simulink model "WaterRunner_open"  (Simulink 8.0)
settings: Solver=ode15s  StartTime=0.0  StopTime=10  FixedStep=1e-3  RelTol=1e-3
values from neighbouring files (symbols this model uses):
  frame_inertia = diag([Ix,Iy,Iz])    [SimParam.m]    (also in matlab.mat = [8.0125e-05  0  0; 0  0.000390625  0; 0  0  0.0003145]; simParams.m; simParams_closed.m; speed_cg.mat = [8.0125e-05  0  0; 0  0.000390625  0; 0  0  0.0003145])
  frame_mass = 0.06    [matlab.mat]    (also in simParam.m = 0.03; simParams.m; simParams_closed.m = 0.1; speed_cg.mat)
  freq = 60    [SimParam.m]    (also in simParam.m = 20; simParams_closed.m)
  L2_inertia = [1.05087286587e-08  0  0; 0  0  0; 0  0  1.05087286587e-08]    [matlab.mat]    (also in simParams.m = diag([I 0 I]); simParams_closed.m = diag([I 0 I]); speed_cg.mat)
  L2_mass = 0.0002653496    [matlab.mat]    (also in simParams.m; simParams_closed.m; speed_cg.mat)
  L3_inertia = [4.24507620885e-07  0  0; 0  0  0; 0  0  4.24507620885e-07]    [matlab.mat]    (also in simParams.m = diag([I 0 I]); simParams_closed.m = diag([I 0 I]); speed_cg.mat)
  L3_mass = 0.0009104656    [matlab.mat]    (also in simParams.m; simParams_closed.m; speed_cg.mat)
  L4_inertia = [1.03972444992e-07  0  0; 0  0  0; 0  0  1.03972444992e-07]    [matlab.mat]    (also in simParams.m = diag([I 0 I]); simParams_closed.m = diag([I 0 I]); speed_cg.mat)
  L4_mass = 0.0005696496    [matlab.mat]    (also in simParams.m; simParams_closed.m; speed_cg.mat)
  water_level = 0    [matlab.mat]    (also in simParam.m; simParams.m; simParams_closed.m; speed_cg.mat)
undefined symbols (not defined in the file): cw_FL_HL, cw_FR_FL, cw_FR_HR, cw_HR_HL, FL_HL_lag, FR_FL_lag, FR_HR_lag, HR_HL_lag, initRobHeight
libraries: mblibv1 x17, WaterRunner_lib x14, simulink x1
settings Model: Creator=fumiyaiida  LastModifiedBy=nitisht  SimulationMode=accelerator
settings SolverCC: ZeroCrossControl=DisableAll
settings DataIOCC: SignalLoggingSaveFormat=ModelDataLogs
settings OptimizationCC: InlineInvariantSignals=on  InitFltsAndDblsToZero=on  EfficientMapNaN2IntZero=off  SimCompilerOptimization=On
settings DebuggingCC: SaveWithParameterizedLinksMsg=none  SignalResolutionControl=TryResolveAllWithWarning  SolverPrmCheckMsg=none  MultiTaskDSMMsg=warning  MultiTaskCondExecSysMsg=none  FcnCallInpInsideContextMsg=UseLocalSettings  StrictBusMsg=None
settings HardwareCC: ProdBitPerLong=64  ProdBitPerPointer=64  ProdIntDivRoundTo=Zero  ProdEndianess=LittleEndian  ProdWordSize=64  ProdHWDeviceType=Intel->x86-64  TargetBitPerLong=64  TargetBitPerPointer=64  TargetIntDivRoundTo=Zero  TargetEndianess=LittleEndian  TargetWordSize=64  TargetHWDeviceType=MATLAB Host  ProdEqTarget=off
settings RTWCC: RTWCompilerOptimization=On
settings CodeAppCC: MaxIdLength=128
settings GRTTargetCC: CombineOutputUpdateFcns=off  GRTInterface=on
settings SimMechanicsCC: WarnOnSingularInitialAssembly=on  VisDuringSimulation=on  VisSampleTime=0.001  AnimationDelay=1  LastVizWinPosition=[1323 2 597 976]  CamPosition=[-7.43826;3.54067;9.27536;]  CamTarget=[0.848137;-0.562095;-0.541519;]  CamUpVector=[0.217493;0.952228;-0.21438;]  CamHeight=2.55  VisBackgroundColor=[0.9;0.9;0.95;]  DefaultBodyColor=[1;0;0;]
settings ConfigurationSet: Description=SimMechanics 2G

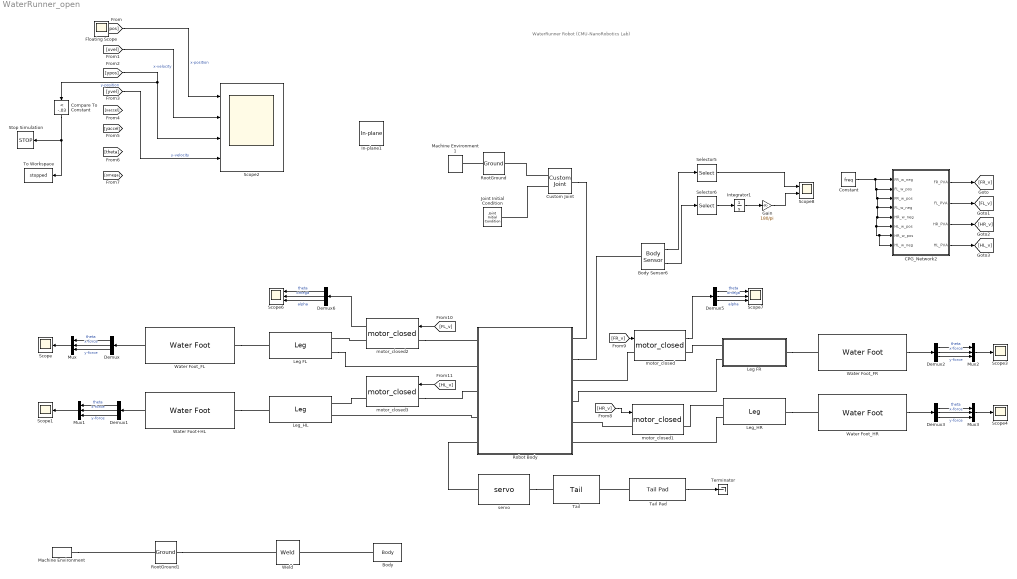
== system WaterRunner_open ==
  note: WaterRunner Robot
      | (CMU-NanoRobotics Lab)
  Body : mblibv1/Bodies/Body  LConnTagsString=CG  UpdateFromCAD=off  DialogClass=MechanicalBodyBlock  Mass=1  MassUnits=kg  InertiaUnits=kg*m^2  Inertia=eye(3)  Shape=Cylinder  ShapeDims=[1 1]  ShapeUnits=m  ShapeUse=false  Density=1  DensityUnits=kg/m^3  DensityUse=false  GraphicsMode=CONVHULL  BodyColorSelMode=COLORPALETTE  BodyColor=[0.83137 0.81569 0.78431]  AttachedToCS=CG  CG=Left$CG$[0 0 0]$WORLD$WORLD$m$[0 0 0]$Euler X-Y-Z$deg$WORLD$true$none  WorkingFrames=Left$CS1$[-0.5 water_level -0.2 ]$CG$CG$m$[0 0 0]$Euler X-Y-Z$deg$WORLD$false$none#Left$CS2$[-0.5 water_level 0.2 ]$CG$CG$m$[0 0 0]$Euler X-Y-Z$deg$WORLD$false$none#Left$CS3$[4 water_level -0.2 ]$CG$CG$m$[0 0 0]$Euler X-Y-Z$deg$WORLD$false$none#Left$CS4$[4 water_level 0.2 ]$CG$CG$m$[0 0 0]$Euler X-Y-Z$deg$WORLD$false$none  CGPos=[0 0 0]  CGRot=[0 0 0]  CS0Pos=[]  CS0Rot=[]  CS1Pos=[-0.5 water_level -0.2 ]  CS1Rot=[0 0 0]  CS2Pos=[-0.5 water_level 0.2 ]  CS2Rot=[0 0 0]  CS3Pos=[4 water_level -0.2 ]  CS3Rot=[0 0 0]  CS4Pos=[4 water_level 0.2 ]  CS4Rot=[0 0 0]  CS5Pos=[]  CS5Rot=[]  CS6Pos=[]  CS6Rot=[]  CS7Pos=[]  CS7Rot=[]  CS8Pos=[]  CS8Rot=[]  CS9Pos=[]  CS9Rot=[]  CS10Pos=[]  CS10Rot=[]  CS11Pos=[]  CS11Rot=[]  CS12Pos=[]  CS12Rot=[]  CS13Pos=[]  CS13Rot=[]  CS14Pos=[]  CS14Rot=[]  CS15Pos=[]  CS15Rot=[]  CS16Pos=[]  CS16Rot=[]  CS17Pos=[]  CS17Rot=[]  CS18Pos=[]  CS18Rot=[]  CS19Pos=[]  CS19Rot=[]  CS20Pos=[]  CS20Rot=[]
  Body Sensor6 : mblibv1/Sensors &  Actuators/Body Sensor  UpdateFromCAD=off  PhysicalDomain=Mechanical  PortType=blob  Muxed=off  Pose=off  Angle=on  AngleUnits=deg  ArcVelocity=on  ArcVelocityUnits=rad/s  ArcAcceleration=off  ArcAccelerationUnits=deg/s^2  CoordPosition=off  CoordPositionUnits=m  Velocity=on  VelocityUnits=m/s  Acceleration=off  AccelerationUnits=m/s^2  Quaternion=on  QuaternionDT=off  QuaternionDDT=off  QuaternionUnits=off  OutputVector=[1]  ActiveIO=on  Width=6  DialogClass=MechanicalSensorBlock  ReferenceFrame=Absolute (World)
  CPG_Network2 : Subsystem
  Compare To Constant : simulink/Logic and Bit Operations/Compare To Constant  relop=<  const=-.03  OutDataTypeStr=boolean
  Constant : Constant  Value=freq
  Custom Joint : mblibv1/Joints/Custom Joint  LConnTagsString=__newl0|SA1  RConnTagsString=__newr0  UpdateFromCAD=off  NumSAPorts=1  CutJoint=off  MarkAsCut=off  Primitives=prismatic  PrimitiveProps=P1$World$[0 1 0]$Prismatic#P2$World$[1 0 0]$Prismatic#R1$World$[0 0 1]$Revolute  DialogClass=JointBlock  R1Axis=[0 0 1]  R2Axis=[]  R3Axis=[]  P1Axis=[0 1 0]  P2Axis=[1 0 0]  P3Axis=[]  SAxis=[]
  Demux{,1..3,5..6} (6 alike) : Demux  Outputs=3
  Gain : Gain  Gain=180/pi
  In-plane1 : mblibv1/Joints/In-plane  LConnTagsString=__newl0|SA1|SA2  RConnTagsString=__newr0|SA1|SA2  UpdateFromCAD=off  NumSAPorts=4  CutJoint=off  MarkAsCut=off  Primitives=prismatic  PrimitiveProps=P1$World$[1 0 0]$prismatic#P2$World$[0 1 0]$prismatic  DialogClass=JointBlock  P1Axis=[1 0 0]  P2Axis=[0 1 0]
  Integrator1 : Integrator
  Joint Initial Condition : mblibv1/Sensors &  Actuators/Joint Initial Condition  UpdateFromCAD=off  LeftPortType=blob  RightPortType=blob  PhysicalDomain=mechanical  DialogClass=InitialConditionBlock  InitialConditions=P1$true$0$m$deg$0$m/s$deg/s#P2$true$initRobHeight$m$deg$0$m/s$deg/s#P3$false$0$m$deg$0$m/s$deg/s#R1$true$0$m$rad$0$m/s$rad/s#R2$false$0$m$deg$0$m/s$deg/s#R3$false$0$m$deg$0$m/s$deg/s#S$false$0$m$deg$0$m/s$deg/s  P1PIC=0  P1VIC=0  P2PIC=initRobHeight  P2VIC=0  P3PIC=0  P3VIC=0  R1PIC=0  R1VIC=0  R2PIC=0  R2VIC=0  R3PIC=0  R3VIC=0  SPIC=0  SVIC=0
  Leg FL : WaterRunner_lib/Leg
  Leg FR : Subsystem  AncestorBlock=WaterRunner_lib/Leg
      mask help: mask for leg
  Leg_HL : WaterRunner_lib/Leg
  Leg_HR : WaterRunner_lib/Leg
  Machine Environment : mblibv1/Bodies/Machine Environment  PortType=env  PhysicalDomain=Mechanical  DialogTemplateClass=MECH.MachineEnvironment  SyncWhenCopied=off  Gravity=[0 -9.81 0]  GravityUnits=m/s^2  GravityAsSignal=off  Dimensionality=Auto-detect  AnalysisType=Forward dynamics  LinearAssemblyTolerance=1e-3  LinearAssemblyToleranceUnits=m  AngularAssemblyTolerance=1e-3  AngularAssemblyToleranceUnits=rad  ConstraintSolverType=Stabilizing  ConstraintRelTolerance=1e-4  ConstraintAbsTolerance=1e-4  UseRobustSingularityHandling=off  RedundancyAnalysisToleranceType=Automatically select tolerance  RedundancyAnalysisTolerance=1e-14  StatePerturbationType=Fixed  PerturbationSize=1e-5  VisualizeMachine=on  BodyVisualizationType=Use model default body geometries  BodyColorSelMode=Use model default  DefaultBodyColor=[1 0 0]
  Machine Environment1 : mblibv1/Bodies/Machine Environment  PortType=env  PhysicalDomain=Mechanical  DialogTemplateClass=MECH.MachineEnvironment  SyncWhenCopied=off  Gravity=[0 -9.81 0]  GravityUnits=m/s^2  GravityAsSignal=off  Dimensionality=Auto-detect  AnalysisType=Forward dynamics  LinearAssemblyTolerance=1e-3  LinearAssemblyToleranceUnits=m  AngularAssemblyTolerance=1e-3  AngularAssemblyToleranceUnits=rad  ConstraintSolverType=Stabilizing  ConstraintRelTolerance=1e-4  ConstraintAbsTolerance=1e-4  UseRobustSingularityHandling=off  RedundancyAnalysisToleranceType=Automatically select tolerance  RedundancyAnalysisTolerance=1e-14  StatePerturbationType=Fixed  PerturbationSize=1e-5  VisualizeMachine=on  BodyVisualizationType=Use model default body geometries  BodyColorSelMode=Use model default  DefaultBodyColor=[1 0 0]
  Mux{,1..3} (4 alike) : Mux  Inputs=3
  Robot Body : Subsystem  AncestorBlock=WaterRunner_lib/Robot Body  mask{initRobHeight=initRobHeight}
      mask prompts: initRobHeight "height"
  RootGround : mblibv1/Bodies/Ground  UpdateFromCAD=on  LeftPortType=env  RightPortType=workingframe  PhysicalDomain=Mechanical  DialogClass=GroundBlock  CoordPosition=[0 0 0]  CoordPositionUnits=m  StateVectorMgrId=1  MachineId=[1 2]  ShowEnvPort=on
  RootGround1 : mblibv1/Bodies/Ground  UpdateFromCAD=on  LeftPortType=env  RightPortType=workingframe  PhysicalDomain=Mechanical  DialogClass=GroundBlock  CoordPosition=[0 0 0]  CoordPositionUnits=m  StateVectorMgrId=0  MachineId=[1 1]  ShowEnvPort=on
  Scope{,1,3..4} (4 alike) : Scope
      Scope settings: ShowLegends=on  TimeRange=2  YMin=-2.5  YMax=2  SaveName=FootForce_FL
      Scope1 settings: ShowLegends=on  TimeRange=2  YMin=-2.5  YMax=2  SaveName=FootForce_HL
      Scope3 settings: ShowLegends=on  TimeRange=2  YMin=-2.5  YMax=2  SaveName=FootForce_FR
      Scope4 settings: ShowLegends=on  TimeRange=2  YMin=-2.5  YMax=2  SaveName=FootForce_HR
  Scope2 : Scope  NumInputPorts=4
      settings: ShowLegends=on  TimeRange=10  YMin=-0.25~0~-0.005~-0.3  YMax=2~2.5~0.035~0.4  SaveName=position
  Scope6 : Scope  NumInputPorts=3
      settings: TimeRange=2  YMin=-20~-90~-50000  YMax=-2.5~0~30000  SaveName=MotorMotion1
  Scope7 : Scope  NumInputPorts=3
      settings: TimeRange=2  YMin=-17.5~-90~-70000  YMax=0~0~30000  SaveName=MotorMotion
  Scope8 : Scope  NumInputPorts=2
      settings: TimeRange=10  YMin=-0.15~0  YMax=0.225~20  SaveName=ball_position
  Selector5 : Selector  InputPortWidth=3  IndexOptions=Index vector (dialog)  Indices=[2]  OutputSizes=1
  Selector6 : Selector  InputPortWidth=3  IndexOptions=Index vector (dialog)  Indices=[1 3]  OutputSizes=1
  Stop Simulation : Stop
  Tail : WaterRunner_lib/Tail
  Tail Pad : WaterRunner_lib/Tail Pad
  Terminator : Terminator
  To Workspace : ToWorkspace  VariableName=stopped  SampleTime=-1  SaveFormat=Timeseries
  Water Foot+HL : WaterRunner_lib/Water Foot
  Water Foot_FL : WaterRunner_lib/Water Foot
  Water Foot_FR : WaterRunner_lib/Water Foot
  Water Foot_HR : WaterRunner_lib/Water Foot
  Weld : mblibv1/Joints/Weld  LConnTagsString=__newl0  RConnTagsString=__newr0  UpdateFromCAD=off  NumSAPorts=0  CutJoint=off  MarkAsCut=off  Primitives=weld  PrimitiveProps=W$WORLD$[0 0 0]$weld  DialogClass=JointBlock  WAxis=[0 0 0]
  motor_closed : WaterRunner_lib/motor_closed  ic_angle=pi
  motor_closed1 : WaterRunner_lib/motor_closed  ic_angle=0
  motor_closed2 : WaterRunner_lib/motor_closed  ic_angle=0
  motor_closed3 : WaterRunner_lib/motor_closed  ic_angle=pi
  servo : WaterRunner_lib/servo  tail_angle=tail_angle  VariableName=work_tail
  Floating Scope : Scope
      settings: Floating=on
  wires:
  Water Foot_FL/1 -> Demux/1
  Demux/1 -> Mux/1  "theta"
  Demux/2 -> Mux/2  "x-force"
  Demux/3 -> Mux/3  "y-force"
  Mux/1 -> Scope/1
  [ypos] -> Compare To Constant/1, Scope2/3  "y-position"
  Water Foot+HL/1 -> Demux1/1
  Demux1/1 -> Mux1/1  "theta"
  Demux1/2 -> Mux1/2  "x-force"
  Demux1/3 -> Mux1/3  "y-force"
  Mux1/1 -> Scope1/1
  Mux2/1 -> Scope3/1
  Demux2/3 -> Mux2/3  "y-force"
  Demux2/2 -> Mux2/2  "x-force"
  Demux2/1 -> Mux2/1  "theta"
  Water Foot_FR/1 -> Demux2/1
  Mux3/1 -> Scope4/1
  Demux3/3 -> Mux3/3  "y-force"
  Demux3/2 -> Mux3/2  "x-force"
  Demux3/1 -> Mux3/1  "theta"
  Water Foot_HR/1 -> Demux3/1
  Compare To Constant/1 -> To Workspace/1, Stop Simulation/1
  Demux5/3 -> Scope7/3  "alpha"
  Demux5/2 -> Scope7/2  "omega"
  Demux5/1 -> Scope7/1  "theta"
  motor_closed/1 -> Demux5/1
  Demux6/3 -> Scope6/3  "alpha"
  Demux6/2 -> Scope6/2  "omega"
  Demux6/1 -> Scope6/1  "theta"
  motor_closed2/1 -> Demux6/1
  Tail Pad/1 -> Terminator/1
  [xpos] -> Scope2/1  "x-position"
  [xvel] -> Scope2/2  "x-velocity"
  [yvel] -> Scope2/4  "y-velocity"
  CPG_Network2/1(FR_PVA) -> [FR_v]
  CPG_Network2/2(FL_PVA) -> [FL_v]
  CPG_Network2/3(HR_PVA) -> [HR_v]
  CPG_Network2/4(HL_PVA) -> [HL_v]
  [FR_v] -> motor_closed/1
  [HR_v] -> motor_closed1/1
  [FL_v] -> motor_closed2/1
  [HL_v] -> motor_closed3/1
  Selector6/1 -> Integrator1/1
  Body Sensor6/2 -> Selector6/1
  Integrator1/1 -> Gain/1
  Gain/1 -> Scope8/2
  Body Sensor6/1 -> Selector5/1
  Selector5/1 -> Scope8/1
  Constant/1 -> CPG_Network2/8(HL_w_neg), CPG_Network2/7(HR_w_pos), CPG_Network2/6(HL_w_pos), CPG_Network2/5(HR_w_neg), CPG_Network2/4(FL_w_neg), CPG_Network2/3(FR_w_pos), CPG_Network2/2(FL_w_pos), CPG_Network2/1(FR_w_neg)
  connections:
  RootGround1/RConn1 -- Weld/LConn1
  Body/LConn1 -- Weld/RConn1
  motor_closed/LConn1 -- Robot Body/RConn3
  Leg FR/LConn2 -- Robot Body/RConn4
  motor_closed/RConn1 -- Leg FR/LConn1
  motor_closed1/LConn1 -- Robot Body/RConn5
  motor_closed1/RConn1 -- Leg_HR/LConn1
  Leg_HR/LConn2 -- Robot Body/RConn6
  Water Foot+HL/LConn1 -- Leg_HL/RConn1
  Water Foot_FL/LConn1 -- Leg FL/RConn1
  Robot Body/LConn4 -- Leg_HL/LConn2
  Leg FR/RConn1 -- Water Foot_FR/LConn1
  Leg_HR/RConn1 -- Water Foot_HR/LConn1
  motor_closed2/LConn1 -- Robot Body/LConn1
  motor_closed3/RConn1 -- Leg_HL/LConn1
  motor_closed3/LConn1 -- Robot Body/LConn3
  Leg FL/LConn2 -- Robot Body/LConn2
  Machine Environment/RConn1 -- RootGround1/LConn1
  motor_closed2/RConn1 -- Leg FL/LConn1
  Robot Body/LConn5 -- servo/LConn1
  servo/RConn1 -- Tail/LConn1
  Tail Pad/LConn1 -- Tail/RConn1
  Custom Joint/LConn1 -- RootGround/RConn1
  Custom Joint/LConn2 -- Joint Initial Condition/RConn1
  RootGround/LConn1 -- Machine Environment1/RConn1
  Robot Body/RConn2 -- Body Sensor6/LConn1
  Custom Joint/RConn1 -- Robot Body/RConn1

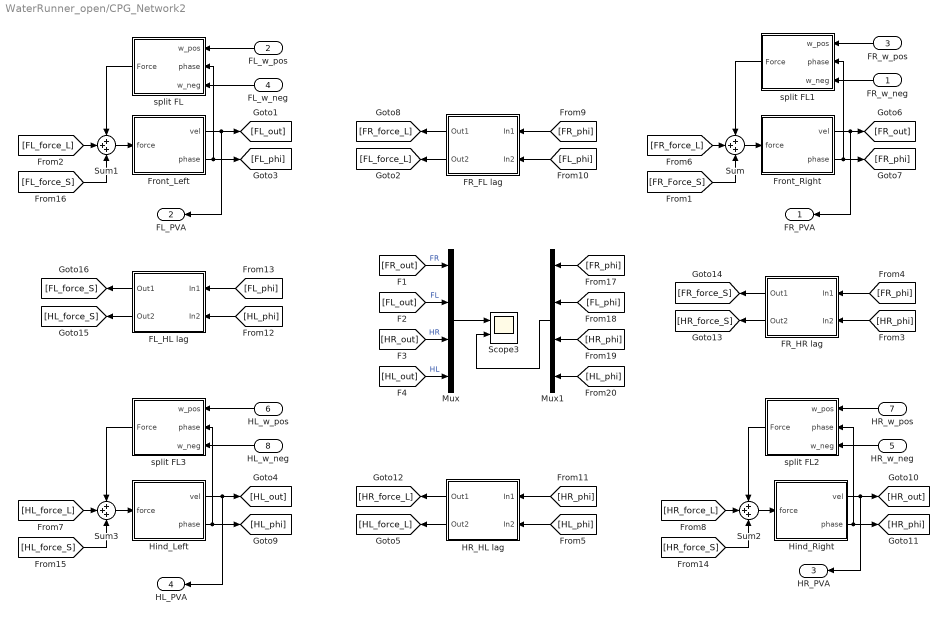
== system WaterRunner_open/CPG_Network2 ==
  FR_w_neg : Inport
  FL_w_pos : Inport  Port=2
  FR_w_pos : Inport  Port=3
  FL_w_neg : Inport  Port=4
  HR_w_neg : Inport  Port=5
  HL_w_pos : Inport  Port=6
  HR_w_pos : Inport  Port=7
  HL_w_neg : Inport  Port=8
  FL_HL lag : Subsystem  mask{d_phase=FL_HL_lag, coupling_weight=cw_FL_HL}
      mask prompts: d_phase "Phase Lag"; coupling_weight "Coupling Weight"
  FR_FL lag : Subsystem  mask{d_phase=FR_FL_lag, coupling_weight=cw_FR_FL}
      mask prompts: d_phase "Phase Lag"; coupling_weight "Coupling Weight"
  FR_HR lag : Subsystem  mask{d_phase=FR_HR_lag, coupling_weight=cw_FR_HR}
      mask prompts: d_phase "Phase Lag"; coupling_weight "Coupling Weight"
  Front_Left : Subsystem  mask{init_phi=0}
      mask prompts: init_phi "Initial Phase"
  Front_Right : Subsystem  mask{init_phi=pi}
      mask prompts: init_phi "Initial Phase"
  HR_HL lag : Subsystem  mask{d_phase=HR_HL_lag, coupling_weight=cw_HR_HL}
      mask prompts: d_phase "Phase Lag"; coupling_weight "Coupling Weight"
  Hind_Left : Subsystem  mask{init_phi=pi}
      mask prompts: init_phi "Initial Phase"
  Hind_Right : Subsystem  mask{init_phi=0}
      mask prompts: init_phi "Initial Phase"
  Mux : Mux
  Mux1 : Mux
  Scope3 : Scope  NumInputPorts=2
      settings: ShowLegends=on  TimeRange=5  YMin=22.11~0  YMax=22.34~6.5  SaveName=Output
  Sum{,1..3} (4 alike) : Sum  Inputs=+++
  split FL : Subsystem
  split FL1 : Subsystem
  split FL2 : Subsystem
  split FL3 : Subsystem
  FR_PVA : Outport
  FL_PVA : Outport  Port=2
  HR_PVA : Outport  Port=3
  HL_PVA : Outport  Port=4
  wires:
  Mux/1 -> Scope3/1
  Front_Left/2(phase) -> split FL/2(phase), [FL_phi]
  Front_Right/2(phase) -> split FL1/2(phase), [FR_phi]
  [FL_phi] -> FR_FL lag/2(In2)
  [FR_phi] -> FR_FL lag/1(In1)
  FR_FL lag/1(Out1) -> [FR_force_L]
  FR_FL lag/2(Out2) -> [FL_force_L]
  Front_Right/1(vel) -> FR_PVA/1, [FR_out]
  [FL_force_L] -> Sum1/2
  Sum1/1 -> Front_Left/1(force)
  Sum/1 -> Front_Right/1(force)
  [FR_force_L] -> Sum/2
  [FL_out] -> Mux/2  "FL"
  [FR_out] -> Mux/1  "FR"
  FR_w_pos/1 -> split FL1/1(w_pos)
  FR_w_neg/1 -> split FL1/3(w_neg)
  split FL1/1(Force) -> Sum/1
  FL_w_pos/1 -> split FL/1(w_pos)
  FL_w_neg/1 -> split FL/3(w_neg)
  Front_Left/1(vel) -> FL_PVA/1, [FL_out]
  split FL/1(Force) -> Sum1/1
  Hind_Left/2(phase) -> split FL3/2(phase), [HL_phi]
  Hind_Right/2(phase) -> [HR_phi], split FL2/2(phase)
  [HL_phi] -> HR_HL lag/2(In2)
  [HR_phi] -> HR_HL lag/1(In1)
  HR_HL lag/1(Out1) -> [HR_force_L]
  HR_HL lag/2(Out2) -> [HL_force_L]
  Hind_Right/1(vel) -> HR_PVA/1, [HR_out]
  [HL_force_L] -> Sum3/2
  Sum3/1 -> Hind_Left/1(force)
  Sum2/1 -> Hind_Right/1(force)
  [HR_force_L] -> Sum2/2
  HR_w_pos/1 -> split FL2/1(w_pos)
  HR_w_neg/1 -> split FL2/3(w_neg)
  split FL2/1(Force) -> Sum2/1
  HL_w_pos/1 -> split FL3/1(w_pos)
  HL_w_neg/1 -> split FL3/3(w_neg)
  Hind_Left/1(vel) -> HL_PVA/1, [HL_out]
  split FL3/1(Force) -> Sum3/1
  [HR_phi] -> FR_HR lag/2(In2)
  [FR_phi] -> FR_HR lag/1(In1)
  FR_HR lag/1(Out1) -> [FR_force_S]
  FR_HR lag/2(Out2) -> [HR_force_S]
  [HL_phi] -> FL_HL lag/2(In2)
  [FL_phi] -> FL_HL lag/1(In1)
  FL_HL lag/1(Out1) -> [FL_force_S]
  FL_HL lag/2(Out2) -> [HL_force_S]
  [HL_out] -> Mux/4  "HL"
  [HR_out] -> Mux/3  "HR"
  [FR_Force_S] -> Sum/3
  [HR_force_S] -> Sum2/3
  [HL_force_S] -> Sum3/3
  [FL_force_S] -> Sum1/3
  Mux1/1 -> Scope3/2
  [FR_phi] -> Mux1/1
  [FL_phi] -> Mux1/2
  [HR_phi] -> Mux1/3
  [HL_phi] -> Mux1/4

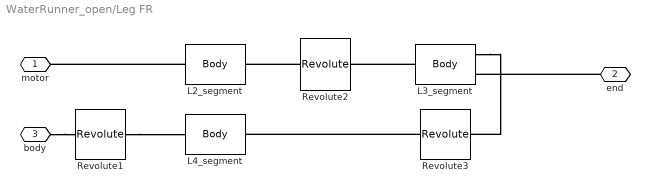
== system WaterRunner_open/Leg FR ==
  L2_segment : mblibv1/Bodies/Body  LConnTagsString=CS1  RConnTagsString=CS2  UpdateFromCAD=off  DialogClass=MechanicalBodyBlock  Mass=L2_mass  MassUnits=kg  InertiaUnits=kg*m^2  Inertia=L2_inertia  Shape=Cylinder  ShapeDims=[1 1]  ShapeUnits=m  ShapeUse=false  Density=1  DensityUnits=kg/m^3  DensityUse=false  GraphicsMode=CONVHULL  BodyColorSelMode=COLORPALETTE  BodyColor=[0 0 0]  AttachedToCS=CG  CG=Left$CG$L2_CG$CS1$CS1$m$[0 0 0]$Euler X-Y-Z$deg$WORLD$false$none  WorkingFrames=Left$CS1$L2_CS1$Adjoining$Adjoining$m$[0 0 0]$Euler X-Y-Z$deg$WORLD$true$none#Right$CS2$L2_CS2$CS1$CS1$m$[0 0 0]$Euler X-Y-Z$deg$WORLD$true$none  CGPos=L2_CG  CGRot=[0 0 0]  CS0Pos=[]  CS0Rot=[]  CS1Pos=L2_CS1  CS1Rot=[0 0 0]  CS2Pos=L2_CS2  CS2Rot=[0 0 0]  CS3Pos=[]  CS3Rot=[]  CS4Pos=[]  CS4Rot=[]  CS5Pos=[]  CS5Rot=[]  CS6Pos=[]  CS6Rot=[]  CS7Pos=[]  CS7Rot=[]  CS8Pos=[]  CS8Rot=[]  CS9Pos=[]  CS9Rot=[]  CS10Pos=[]  CS10Rot=[]  CS11Pos=[]  CS11Rot=[]  CS12Pos=[]  CS12Rot=[]  CS13Pos=[]  CS13Rot=[]  CS14Pos=[]  CS14Rot=[]  CS15Pos=[]  CS15Rot=[]  CS16Pos=[]  CS16Rot=[]  CS17Pos=[]  CS17Rot=[]  CS18Pos=[]  CS18Rot=[]  CS19Pos=[]  CS19Rot=[]  CS20Pos=[]  CS20Rot=[]
  L3_segment : mblibv1/Bodies/Body  LConnTagsString=CS1  RConnTagsString=CS2|CS3  UpdateFromCAD=off  DialogClass=MechanicalBodyBlock  Mass=L3_mass  MassUnits=kg  InertiaUnits=kg*m^2  Inertia=L3_inertia  Shape=Cylinder  ShapeDims=[1 1]  ShapeUnits=m  ShapeUse=false  Density=1  DensityUnits=kg/m^3  DensityUse=false  GraphicsMode=CONVHULL  BodyColorSelMode=COLORPALETTE  BodyColor=[0 0 0]  AttachedToCS=CG  CG=Left$CG$L3_CG$CS1$CS1$m$[0 0 0]$Euler X-Y-Z$rad$CS1$false$none  WorkingFrames=Left$CS1$L3_CS1$Adjoining$Adjoining$m$L3_ori$Euler X-Y-Z$rad$Adjoining$true$none#Right$CS2$L3_CS2$CS1$CS1$m$[0 0 0]$Euler X-Y-Z$rad$CS1$true$none#Right$CS3$L3_CS3$CS1$CS1$m$[0 0 0]$Euler X-Y-Z$rad$CS1$true$none  CGPos=L3_CG  CGRot=[0 0 0]  CS0Pos=[]  CS0Rot=[]  CS1Pos=L3_CS1  CS1Rot=L3_ori  CS2Pos=L3_CS2  CS2Rot=[0 0 0]  CS3Pos=L3_CS3  CS3Rot=[0 0 0]  CS4Pos=[]  CS4Rot=[]  CS5Pos=[]  CS5Rot=[]  CS6Pos=[]  CS6Rot=[]  CS7Pos=[]  CS7Rot=[]  CS8Pos=[]  CS8Rot=[]  CS9Pos=[]  CS9Rot=[]  CS10Pos=[]  CS10Rot=[]  CS11Pos=[]  CS11Rot=[]  CS12Pos=[]  CS12Rot=[]  CS13Pos=[]  CS13Rot=[]  CS14Pos=[]  CS14Rot=[]  CS15Pos=[]  CS15Rot=[]  CS16Pos=[]  CS16Rot=[]  CS17Pos=[]  CS17Rot=[]  CS18Pos=[]  CS18Rot=[]  CS19Pos=[]  CS19Rot=[]  CS20Pos=[]  CS20Rot=[]
  L4_segment : mblibv1/Bodies/Body  LConnTagsString=CS1  RConnTagsString=CS2  UpdateFromCAD=off  DialogClass=MechanicalBodyBlock  Mass=L4_mass  MassUnits=kg  InertiaUnits=kg*m^2  Inertia=L4_inertia  Shape=Cylinder  ShapeDims=[1 1]  ShapeUnits=m  ShapeUse=false  Density=1  DensityUnits=kg/m^3  DensityUse=false  GraphicsMode=CONVHULL  BodyColorSelMode=COLORPALETTE  BodyColor=[0 0 0]  AttachedToCS=CG  CG=Left$CG$L4_CG$CS1$CS1$m$[0 0 0]$Euler X-Y-Z$rad$CS1$false$none  WorkingFrames=Left$CS1$L4_CS1$Adjoining$Adjoining$m$L4_ori$Euler X-Y-Z$rad$Adjoining$true$none#Right$CS2$L4_CS2$CS1$CS1$m$[0 0 0]$Euler X-Y-Z$rad$CS1$true$none  CGPos=L4_CG  CGRot=[0 0 0]  CS0Pos=[]  CS0Rot=[]  CS1Pos=L4_CS1  CS1Rot=L4_ori  CS2Pos=L4_CS2  CS2Rot=[0 0 0]  CS3Pos=[]  CS3Rot=[]  CS4Pos=[]  CS4Rot=[]  CS5Pos=[]  CS5Rot=[]  CS6Pos=[]  CS6Rot=[]  CS7Pos=[]  CS7Rot=[]  CS8Pos=[]  CS8Rot=[]  CS9Pos=[]  CS9Rot=[]  CS10Pos=[]  CS10Rot=[]  CS11Pos=[]  CS11Rot=[]  CS12Pos=[]  CS12Rot=[]  CS13Pos=[]  CS13Rot=[]  CS14Pos=[]  CS14Rot=[]  CS15Pos=[]  CS15Rot=[]  CS16Pos=[]  CS16Rot=[]  CS17Pos=[]  CS17Rot=[]  CS18Pos=[]  CS18Rot=[]  CS19Pos=[]  CS19Rot=[]  CS20Pos=[]  CS20Rot=[]
  Revolute1 : mblibv1/Joints/Revolute  LConnTagsString=__newl0  RConnTagsString=__newr0  UpdateFromCAD=off  NumSAPorts=0  CutJoint=off  MarkAsCut=off  Primitives=prismatic  PrimitiveProps=R1$World$[0 0 1]$revolute  DialogClass=JointBlock  R1Axis=[0 0 1]
  Revolute2 : mblibv1/Joints/Revolute  LConnTagsString=__newl0  RConnTagsString=__newr0  UpdateFromCAD=off  NumSAPorts=0  CutJoint=on  MarkAsCut=off  Primitives=prismatic  PrimitiveProps=R1$World$[0 0 1]$revolute  DialogClass=JointBlock  R1Axis=[0 0 1]
  Revolute3 : mblibv1/Joints/Revolute  LConnTagsString=__newl0  RConnTagsString=__newr0  UpdateFromCAD=off  NumSAPorts=0  CutJoint=off  MarkAsCut=off  Primitives=prismatic  PrimitiveProps=R1$World$[0 0 1]$revolute  DialogClass=JointBlock  R1Axis=[0 0 1]
  motor : PMIOPort  Port=1  Side=Left
  end : PMIOPort  Port=2  Side=Right
  body : PMIOPort  Port=3  Side=Left
  connections:
  L2_segment/LConn1 -- motor/RConn1
  Revolute2/LConn1 -- L2_segment/RConn1
  L3_segment/LConn1 -- Revolute2/RConn1
  L3_segment/RConn1 -- Revolute3/RConn1
  Revolute1/RConn1 -- L4_segment/LConn1
  Revolute3/LConn1 -- L4_segment/RConn1
  body/RConn1 -- Revolute1/LConn1
  end/RConn1 -- L3_segment/RConn2

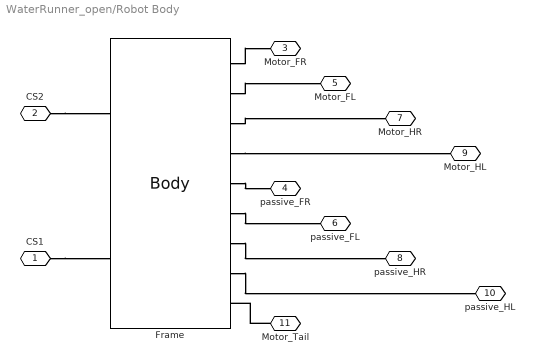
== system WaterRunner_open/Robot Body ==
  Frame : mblibv1/Bodies/Body  LConnTagsString=CG|CS1  RConnTagsString=CS6|CS7|CS8|CS9|CS10|CS11|CS12|CS13|CS14  UpdateFromCAD=off  DialogClass=MechanicalBodyBlock  Mass=frame_mass  MassUnits=kg  InertiaUnits=kg*m^2  Inertia=frame_inertia  Shape=Cylinder  ShapeDims=[1 1]  ShapeUnits=m  ShapeUse=false  Density=1  DensityUnits=kg/m^3  DensityUse=false  GraphicsMode=CONVHULL  BodyColorSelMode=COLORPALETTE  BodyColor=[0 0 1]  AttachedToCS=CG  CG=Left$CG$frame_CG$WORLD$WORLD$m$[0 0 0]$Euler X-Y-Z$deg$WORLD$true$none  WorkingFrames=Left$CS1$frame_CA$World$World$m$[0 0 0]$Euler X-Y-Z$deg$WORLD$true$none#Right$CS2$frame_FR$World$World$m$[0 0 0]$Euler X-Y-Z$deg$WORLD$false$none#Right$CS4$frame_FL$World$World$m$[0 0 0]$Euler X-Y-Z$deg$WORLD$false$none#Right$CS3$frame_HR$World$World$m$[0 0 0]$Euler X-Y-Z$deg$WORLD$false$none#Right$CS5$frame_HL$WORLD$WORLD$m$[0 0 0]$Euler X-Y-Z$deg$WORLD$false$none#Right$CS6$frame_motor_FR$WORLD$WORLD$m$[0 0 0]$Euler X-Y-Z$deg$WORLD$true$none#Right$CS7$frame_motor_FL$WORLD$WORLD$m$[0 0 0]$Euler X-Y-Z$deg$WORLD$true$none#Right$CS8$frame_motor_HR$WORLD$WORLD$m$[0 0 0]$Euler X-Y-Z$deg$WORLD$true$none#Right$CS9$frame_motor_HL$WORLD$WORLD$m$[0 0 0]$Euler X-Y-Z$deg$WORLD$true$none#Right$CS10$frame_passive_FR$WORLD$WORLD$m$[0 0 0]$Euler X-Y-Z$deg$WORLD$true$none#Right$CS11$frame_passive_FL$WORLD$WORLD$m$[0 0 0]$Euler X-Y-Z$deg$WORLD$true$none#Right$CS12$frame_passive_HR$WORLD$WORLD$m$[0 0 0]$Euler X-Y-Z$deg$WORLD$true$none#Right$CS13$frame_passive_HL$WORLD$WORLD$m$[0 0 0]$Euler X-Y-Z$deg$WORLD$true$none#Right$CS14$frame_motor_Tail$WORLD$WORLD$m$[0 0 0]$Euler X-Y-Z$deg$WORLD$true$none  CGPos=frame_CG  CGRot=[0 0 0]  CS0Pos=[]  CS0Rot=[]  CS1Pos=frame_CA  CS1Rot=[0 0 0]  CS2Pos=frame_FR  CS2Rot=[0 0 0]  CS3Pos=frame_HR  CS3Rot=[0 0 0]  CS4Pos=frame_FL  CS4Rot=[0 0 0]  CS5Pos=frame_HL  CS5Rot=[0 0 0]  CS6Pos=frame_motor_FR  CS6Rot=[0 0 0]  CS7Pos=frame_motor_FL  CS7Rot=[0 0 0]  CS8Pos=frame_motor_HR  CS8Rot=[0 0 0]  CS9Pos=frame_motor_HL  CS9Rot=[0 0 0]  CS10Pos=frame_passive_FR  CS10Rot=[0 0 0]  CS11Pos=frame_passive_FL  CS11Rot=[0 0 0]  CS12Pos=frame_passive_HR  CS12Rot=[0 0 0]  CS13Pos=frame_passive_HL  CS13Rot=[0 0 0]  CS14Pos=frame_motor_Tail  CS14Rot=[0 0 0]  CS15Pos=[]  CS15Rot=[]  CS16Pos=[]  CS16Rot=[]  CS17Pos=[]  CS17Rot=[]  CS18Pos=[]  CS18Rot=[]  CS19Pos=[]  CS19Rot=[]  CS20Pos=[]  CS20Rot=[]
  CS1 : PMIOPort  Port=1  Side=Right
  CS2 : PMIOPort  Port=2  Side=Right
  Motor_FR : PMIOPort  Port=3  Side=Right
  passive_FR : PMIOPort  Port=4  Side=Right
  Motor_FL : PMIOPort  Port=5  Side=Left
  passive_FL : PMIOPort  Port=6  Side=Left
  Motor_HR : PMIOPort  Port=7  Side=Right
  passive_HR : PMIOPort  Port=8  Side=Right
  Motor_HL : PMIOPort  Port=9  Side=Left
  passive_HL : PMIOPort  Port=10  Side=Left
  Motor_Tail : PMIOPort  Port=11  Side=Left
  connections:
  Motor_Tail/RConn1 -- Frame/RConn9
  Frame/RConn8 -- passive_HL/RConn1
  Frame/RConn7 -- passive_HR/RConn1
  Frame/RConn6 -- passive_FL/RConn1
  Frame/RConn5 -- passive_FR/RConn1
  Frame/RConn4 -- Motor_HL/RConn1
  Frame/RConn3 -- Motor_HR/RConn1
  Frame/RConn2 -- Motor_FL/RConn1
  Frame/RConn1 -- Motor_FR/RConn1
  CS1/RConn1 -- Frame/LConn2
  CS2/RConn1 -- Frame/LConn1

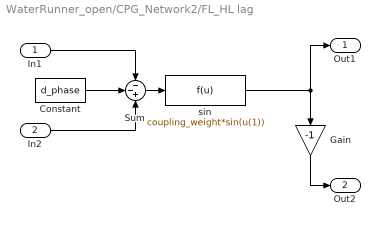
== system WaterRunner_open/CPG_Network2/FL_HL lag ==
  In1 : Inport
  In2 : Inport  Port=2
  Constant : Constant  Value=d_phase
  Gain : Gain  Gain=-1
  Sum : Sum  Inputs=--+
  sin : Fcn  Expr=coupling_weight*sin(u(1))
  Out1 : Outport
  Out2 : Outport  Port=2
  wires:
  Sum/1 -> sin/1
  sin/1 -> Gain/1, Out1/1
  Constant/1 -> Sum/2
  In1/1 -> Sum/1
  In2/1 -> Sum/3
  Gain/1 -> Out2/1

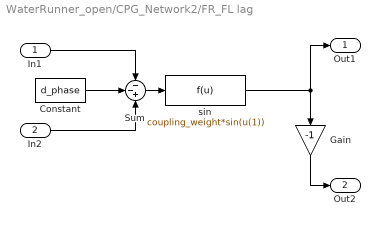
== system WaterRunner_open/CPG_Network2/FR_FL lag ==
  In1 : Inport
  In2 : Inport  Port=2
  Constant : Constant  Value=d_phase
  Gain : Gain  Gain=-1
  Sum : Sum  Inputs=--+
  sin : Fcn  Expr=coupling_weight*sin(u(1))
  Out1 : Outport
  Out2 : Outport  Port=2
  wires:
  Sum/1 -> sin/1
  sin/1 -> Gain/1, Out1/1
  Constant/1 -> Sum/2
  In1/1 -> Sum/1
  In2/1 -> Sum/3
  Gain/1 -> Out2/1

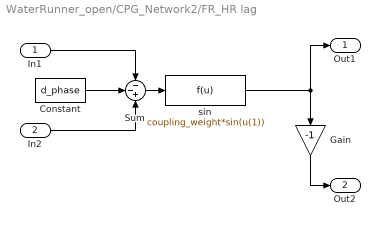
== system WaterRunner_open/CPG_Network2/FR_HR lag ==
  In1 : Inport
  In2 : Inport  Port=2
  Constant : Constant  Value=d_phase
  Gain : Gain  Gain=-1
  Sum : Sum  Inputs=--+
  sin : Fcn  Expr=coupling_weight*sin(u(1))
  Out1 : Outport
  Out2 : Outport  Port=2
  wires:
  Gain/1 -> Out2/1
  In2/1 -> Sum/3
  In1/1 -> Sum/1
  Constant/1 -> Sum/2
  sin/1 -> Out1/1, Gain/1
  Sum/1 -> sin/1

== system WaterRunner_open/CPG_Network2/Front_Left ==
  force : Inport
  Integrator3 : Integrator  InitialCondition=init_phi + 0.001*rand
  Mod 2pi : Fcn  Expr=atan2(sin(u(1)-pi),cos(u(1)-pi))+pi
  vel : Outport
  phase : Outport  Port=2
  wires:
  force/1 -> vel/1, Integrator3/1
  Integrator3/1 -> Mod 2pi/1
  Mod 2pi/1 -> phase/1

== system WaterRunner_open/CPG_Network2/Front_Right ==
  force : Inport
  Integrator3 : Integrator  InitialCondition=init_phi + 0.001*rand
  Mod 2pi : Fcn  Expr=atan2(sin(u(1)-pi),cos(u(1)-pi))+pi
  vel : Outport
  phase : Outport  Port=2
  wires:
  Mod 2pi/1 -> phase/1
  Integrator3/1 -> Mod 2pi/1
  force/1 -> Integrator3/1, vel/1

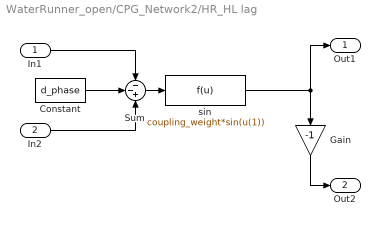
== system WaterRunner_open/CPG_Network2/HR_HL lag ==
  In1 : Inport
  In2 : Inport  Port=2
  Constant : Constant  Value=d_phase
  Gain : Gain  Gain=-1
  Sum : Sum  Inputs=--+
  sin : Fcn  Expr=coupling_weight*sin(u(1))
  Out1 : Outport
  Out2 : Outport  Port=2
  wires:
  Gain/1 -> Out2/1
  In2/1 -> Sum/3
  In1/1 -> Sum/1
  Constant/1 -> Sum/2
  sin/1 -> Out1/1, Gain/1
  Sum/1 -> sin/1

== system WaterRunner_open/CPG_Network2/Hind_Left ==
  force : Inport
  Integrator3 : Integrator  InitialCondition=init_phi + 0.001*rand
  Mod 2pi : Fcn  Expr=atan2(sin(u(1)-pi),cos(u(1)-pi))+pi
  vel : Outport
  phase : Outport  Port=2
  wires:
  force/1 -> vel/1, Integrator3/1
  Integrator3/1 -> Mod 2pi/1
  Mod 2pi/1 -> phase/1

== system WaterRunner_open/CPG_Network2/Hind_Right ==
  force : Inport
  Integrator3 : Integrator  InitialCondition=init_phi + 0.001*rand
  Mod 2pi : Fcn  Expr=atan2(sin(u(1)-pi),cos(u(1)-pi))+pi
  vel : Outport
  phase : Outport  Port=2
  wires:
  force/1 -> vel/1, Integrator3/1
  Integrator3/1 -> Mod 2pi/1
  Mod 2pi/1 -> phase/1

== system WaterRunner_open/CPG_Network2/split FL ==
  w_pos : Inport
  phase : Inport  Port=2
  w_neg : Inport  Port=3
  Product : Product  RndMeth=Zero
  Product1 : Product  RndMeth=Zero
  Sum2 : Sum  Inputs=|++
  enable : Subsystem
  Force : Outport
  wires:
  Product/1 -> Sum2/1
  w_pos/1 -> Product/1
  w_neg/1 -> Product1/1
  Product1/1 -> Sum2/2
  enable/1(pos) -> Product/2
  enable/2(neg) -> Product1/2
  Sum2/1 -> Force/1
  phase/1 -> enable/1(in)

== system WaterRunner_open/CPG_Network2/split FL1 ==
  w_pos : Inport
  phase : Inport  Port=2
  w_neg : Inport  Port=3
  Product : Product  RndMeth=Zero
  Product1 : Product  RndMeth=Zero
  Sum2 : Sum  Inputs=|++
  enable : Subsystem
  Force : Outport
  wires:
  Product/1 -> Sum2/1
  w_pos/1 -> Product/1
  w_neg/1 -> Product1/1
  Product1/1 -> Sum2/2
  enable/1(pos) -> Product/2
  enable/2(neg) -> Product1/2
  Sum2/1 -> Force/1
  phase/1 -> enable/1(in)

== system WaterRunner_open/CPG_Network2/split FL2 ==
  w_pos : Inport
  phase : Inport  Port=2
  w_neg : Inport  Port=3
  Product : Product  RndMeth=Zero
  Product1 : Product  RndMeth=Zero
  Sum2 : Sum  Inputs=|++
  enable : Subsystem
  Force : Outport
  wires:
  phase/1 -> enable/1(in)
  Sum2/1 -> Force/1
  enable/2(neg) -> Product1/2
  enable/1(pos) -> Product/2
  Product1/1 -> Sum2/2
  w_neg/1 -> Product1/1
  w_pos/1 -> Product/1
  Product/1 -> Sum2/1

== system WaterRunner_open/CPG_Network2/split FL3 ==
  w_pos : Inport
  phase : Inport  Port=2
  w_neg : Inport  Port=3
  Product : Product  RndMeth=Zero
  Product1 : Product  RndMeth=Zero
  Sum2 : Sum  Inputs=|++
  enable : Subsystem
  Force : Outport
  wires:
  Product/1 -> Sum2/1
  w_pos/1 -> Product/1
  w_neg/1 -> Product1/1
  Product1/1 -> Sum2/2
  enable/1(pos) -> Product/2
  enable/2(neg) -> Product1/2
  Sum2/1 -> Force/1
  phase/1 -> enable/1(in)

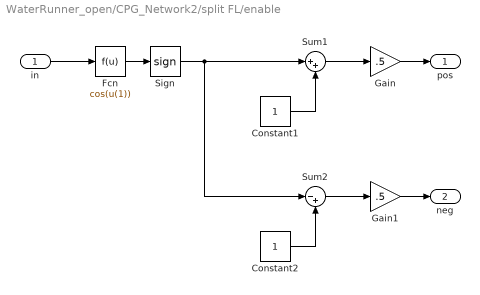
== system WaterRunner_open/CPG_Network2/split FL/enable ==
  in : Inport
  Constant1 : Constant
  Constant2 : Constant
  Fcn : Fcn  Expr=cos(u(1))
  Gain : Gain  Gain=.5
  Gain1 : Gain  Gain=.5
  Sign : Signum
  Sum1 : Sum  Inputs=|++
  Sum2 : Sum  Inputs=|-+
  pos : Outport
  neg : Outport  Port=2
  wires:
  Fcn/1 -> Sign/1
  Constant1/1 -> Sum1/2
  Sign/1 -> Sum2/1, Sum1/1
  Gain/1 -> pos/1
  in/1 -> Fcn/1
  Sum1/1 -> Gain/1
  Constant2/1 -> Sum2/2
  Gain1/1 -> neg/1
  Sum2/1 -> Gain1/1

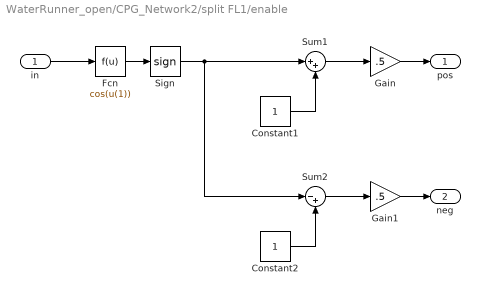
== system WaterRunner_open/CPG_Network2/split FL1/enable ==
  in : Inport
  Constant1 : Constant
  Constant2 : Constant
  Fcn : Fcn  Expr=cos(u(1))
  Gain : Gain  Gain=.5
  Gain1 : Gain  Gain=.5
  Sign : Signum
  Sum1 : Sum  Inputs=|++
  Sum2 : Sum  Inputs=|-+
  pos : Outport
  neg : Outport  Port=2
  wires:
  Fcn/1 -> Sign/1
  Constant1/1 -> Sum1/2
  Sign/1 -> Sum2/1, Sum1/1
  Gain/1 -> pos/1
  in/1 -> Fcn/1
  Sum1/1 -> Gain/1
  Constant2/1 -> Sum2/2
  Gain1/1 -> neg/1
  Sum2/1 -> Gain1/1

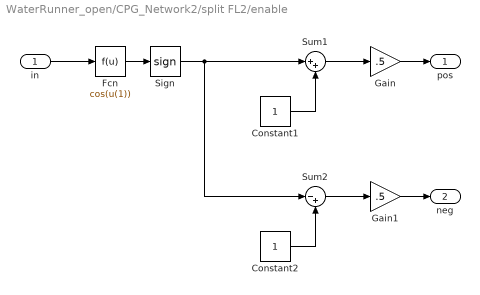
== system WaterRunner_open/CPG_Network2/split FL2/enable ==
  in : Inport
  Constant1 : Constant
  Constant2 : Constant
  Fcn : Fcn  Expr=cos(u(1))
  Gain : Gain  Gain=.5
  Gain1 : Gain  Gain=.5
  Sign : Signum
  Sum1 : Sum  Inputs=|++
  Sum2 : Sum  Inputs=|-+
  pos : Outport
  neg : Outport  Port=2
  wires:
  Sum2/1 -> Gain1/1
  Gain1/1 -> neg/1
  Constant2/1 -> Sum2/2
  Sum1/1 -> Gain/1
  in/1 -> Fcn/1
  Gain/1 -> pos/1
  Sign/1 -> Sum1/1, Sum2/1
  Constant1/1 -> Sum1/2
  Fcn/1 -> Sign/1

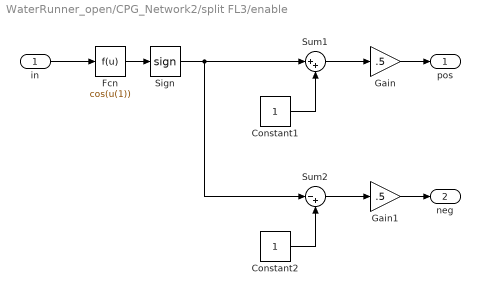
== system WaterRunner_open/CPG_Network2/split FL3/enable ==
  in : Inport
  Constant1 : Constant
  Constant2 : Constant
  Fcn : Fcn  Expr=cos(u(1))
  Gain : Gain  Gain=.5
  Gain1 : Gain  Gain=.5
  Sign : Signum
  Sum1 : Sum  Inputs=|++
  Sum2 : Sum  Inputs=|-+
  pos : Outport
  neg : Outport  Port=2
  wires:
  Fcn/1 -> Sign/1
  Constant1/1 -> Sum1/2
  Sign/1 -> Sum2/1, Sum1/1
  Gain/1 -> pos/1
  in/1 -> Fcn/1
  Sum1/1 -> Gain/1
  Constant2/1 -> Sum2/2
  Gain1/1 -> neg/1
  Sum2/1 -> Gain1/1
